simulink model "SF103A_MotRefMdl"  (R2013b)
settings: Solver=FixedStepDiscrete  StartTime=0.0  StopTime=2  FixedStep=.002  RelTol=1e-3
values from neighbouring files (symbols this model uses):
  ARCHGLBPRM_2MILLISEC_SEC_F32 = DataDict.Constant    [SF103A_MotRefMdl_DataDict.m]
  ARCHGLBPRM_2OVERSQRT3_ULS_F32 = DataDict.Constant    [SF103A_MotRefMdl_DataDict.m]
  ARCHGLBPRM_2PI_ULS_F32 = DataDict.Constant    [SF103A_MotRefMdl_DataDict.m]
  ARCHGLBPRM_4OVERSQRT3_ULS_F32 = DataDict.Constant    [SF103A_MotRefMdl_DataDict.m]
  ARCHGLBPRM_5PIOVER4_ULS_F32 = DataDict.Constant    [SF103A_MotRefMdl_DataDict.m]
  ARCHGLBPRM_FLOATZEROTHD_ULS_F32 = DataDict.Constant    [SF103A_MotRefMdl_DataDict.m]
  ARCHGLBPRM_HALFSQRT3_ULS_F32 = DataDict.Constant    [SF103A_MotRefMdl_DataDict.m]
  ARCHGLBPRM_PI_ULS_F32 = DataDict.Constant    [SF103A_MotRefMdl_DataDict.m]
  MotRefMdlCurrDaxBoostGain = DataDict.Calibration    [SF103A_MotRefMdl_DataDict.m]
  MotRefMdlCurrDaxQaxRefDelta = DataDict.Calibration    [SF103A_MotRefMdl_DataDict.m]
  MotRefMdlCurrItrnTolr = DataDict.Calibration    [SF103A_MotRefMdl_DataDict.m]
  MotRefMdlFbCtrlDi = DataDict.Calibration    [SF103A_MotRefMdl_DataDict.m]
  MotRefMdlIvtrDeadTiBrdgVltgSca = DataDict.Calibration    [SF103A_MotRefMdl_DataDict.m]
  MotRefMdlMinCurrItrnLim = DataDict.Calibration    [SF103A_MotRefMdl_DataDict.m]
  MotRefMdlMotCurrDaxMaxSca = DataDict.Calibration    [SF103A_MotRefMdl_DataDict.m]
  MotRefMdlMotVltgDerivtvTiCon = DataDict.Calibration    [SF103A_MotRefMdl_DataDict.m]
  MotRefMdlRefLocnItrnLim = DataDict.Calibration    [SF103A_MotRefMdl_DataDict.m]
  MotRefMdlTqItrnLim = DataDict.Calibration    [SF103A_MotRefMdl_DataDict.m]
  MotRefMdlTqItrnTolr = DataDict.Calibration    [SF103A_MotRefMdl_DataDict.m]
  MotRefMdlVltgModDynCmpEna = DataDict.Calibration    [SF103A_MotRefMdl_DataDict.m]
  MotRefMdlVltgOverRThdSca = DataDict.Calibration    [SF103A_MotRefMdl_DataDict.m]
  SysGlbPrmMotPoleCnt = DataDict.ImprtdCal    [SF103A_MotRefMdl_DataDict.m]
undefined symbols (not defined in the file or in its folder): MotQuad1
libraries: NxtrLim x18, simulink x4, LnrIntrpn x3, Fil x2, NxtrAbslt x2, FixdToFloat x2, FloatToFixd x2, NxtrMath x1
(part 7 of 7)

== system SF103A_MotRefMdl/MotRefMdl/MotRefMdlPer1/LocateTorqueExtremes/WrapBracketAngles/No_Wrapping ==
  note: NOTE: Zero-based indexing
  TqAry : Inport  RequirementInfo={} %GIDa_95b60389_312e_4e00_baea_f2a06bc6961c
  Idx : Inport  RequirementInfo={} %GIDa_85d3ca93_8505_4e13_896f_eb03525bfb00  Port=2
  Action Port : ActionPort  ActionType=else
  Add : Sum  RequirementInfo="{'linktype_rmi_doors' '0000bb42 (/E-STEER Core/SubSystem Specifications/Application Functions/SF99/SF103A Motor Reference Model)' '#SF103A_138' 'true' 'REQ:  SF103A_138' '' } %GIDa_76d2b924_a1a6_47e1_8dc3_f936241e4074"  Inputs=+-
  Add1 : Sum  RequirementInfo="{'linktype_rmi_doors' '0000bb42 (/E-STEER Core/SubSystem Specifications/Application Functions/SF99/SF103A Motor Reference Model)' '#SF103A_138' 'true' 'REQ:  SF103A_138' '' } %GIDa_2d784fd6_0602_4f9b_a025_1580a0ab04f6"
  Bus Creator : BusCreator  RequirementInfo={} %GIDa_72eb0c74_95b4_429b_92eb_e52945b126cd  Inputs=6
  Constant1 : Constant  RequirementInfo="{'linktype_rmi_doors' '0000bb42 (/E-STEER Core/SubSystem Specifications/Application Functions/SF99/SF103A Motor Reference Model)' '#SF103A_138' 'true' 'REQ:  SF103A_138' '' } %GIDa_ebffaea6_e14f_413b_adce_d0d0bfcaa7a2"  SampleTime=-1
  Constant2 : Constant  RequirementInfo="{'linktype_rmi_doors' '0000bb42 (/E-STEER Core/SubSystem Specifications/Application Functions/SF99/SF103A Motor Reference Model)' '#SF103A_138' 'true' 'REQ:  SF103A_138' '' } %GIDa_04d63c2b_3e97_4bb2_a3c0_64e6c76ecc75"  SampleTime=-1
  Constant6 : Constant  RequirementInfo="{'linktype_rmi_doors' '0000bb42 (/E-STEER Core/SubSystem Specifications/Application Functions/SF99/SF103A Motor Reference Model)' '#SF103A_138' 'true' 'REQ:  SF103A_138' '' } %GIDa_7fe1ae96_fb88_4a92_9eeb_3c5b2c10fb83"  Value=MotRefMdlCurrDaxQaxRefDelta
  CopyRight2 : Subsystem  Description=|  mask(Copyright Information){none=on}
      | Copyright info block.                                               
      |                                                                     
      | Place copyright information at the top of every subsystem in design.
      mask prompts: none "No parameters"
      mask help: Place copyright information at the top of every subsystem in design.
      mask Display:
      | NxtrConf = 'Nexteer Confidential';
      | 
      | sys = bdroot; %handle for the current model ("system")
      | first = get_param(sys,'Created');
      | first = first(end-3:end);  %year is last four digits
      | 
      | last = get_param(sys,'LastModifiedDate');
      | if isempty(last)
      |     last = datestr(now,'yyyy');
      | else
      |     last = last(end-3:end);
      | end
      | 
      | if strcmp(first,last)
      |     fprintf('%s -- Copyright %s Nexteer',NxtrConf,first)
      | else
      |     fprintf('%s -- %s%s- %s Nexteer',NxtrConf,char(169),first,last)
      | end
  Index Vector : MultiPortSwitch  RequirementInfo="{'linktype_rmi_doors' '0000bb42 (/E-STEER Core/SubSystem Specifications/Application Functions/SF99/SF103A Motor Reference Model)' '#SF103A_138' 'true' 'REQ:  SF103A_138' '' } %GIDa_7f96635d_e863_42f7_be0b_d83f99408380"  DataPortOrder=Zero-based contiguous  Inputs=1
  Index Vector1 : MultiPortSwitch  RequirementInfo="{'linktype_rmi_doors' '0000bb42 (/E-STEER Core/SubSystem Specifications/Application Functions/SF99/SF103A Motor Reference Model)' '#SF103A_138' 'true' 'REQ:  SF103A_138' '' } %GIDa_df08fecc_11d0_46ed_8f6c_a3725551e30a"  DataPortOrder=Zero-based contiguous  Inputs=1
  Index Vector2 : MultiPortSwitch  RequirementInfo="{'linktype_rmi_doors' '0000bb42 (/E-STEER Core/SubSystem Specifications/Application Functions/SF99/SF103A Motor Reference Model)' '#SF103A_138' 'true' 'REQ:  SF103A_138' '' } %GIDa_93665409_302c_47f3_aba1_ec404b710aa3"  DataPortOrder=Zero-based contiguous  Inputs=1
  Index Vector3 : MultiPortSwitch  RequirementInfo="{'linktype_rmi_doors' '0000bb42 (/E-STEER Core/SubSystem Specifications/Application Functions/SF99/SF103A Motor Reference Model)' '#SF103A_138' 'true' 'REQ:  SF103A_138' '' } %GIDa_c4c60c45_93ef_41e4_9634_c6d7fcea99cf"  DataPortOrder=Zero-based contiguous  Inputs=1
  Index Vector4 : MultiPortSwitch  RequirementInfo="{'linktype_rmi_doors' '0000bb42 (/E-STEER Core/SubSystem Specifications/Application Functions/SF99/SF103A Motor Reference Model)' '#SF103A_138' 'true' 'REQ:  SF103A_138' '' } %GIDa_24382880_2f97_4ce1_8410_907a3d96e683"  DataPortOrder=Zero-based contiguous  Inputs=1
  Index Vector5 : MultiPortSwitch  RequirementInfo="{'linktype_rmi_doors' '0000bb42 (/E-STEER Core/SubSystem Specifications/Application Functions/SF99/SF103A Motor Reference Model)' '#SF103A_138' 'true' 'REQ:  SF103A_138' '' } %GIDa_8818387d_5b6e_4e1f_aee0_609f703e5b56"  DataPortOrder=Zero-based contiguous  Inputs=1
  IntrpnPts : Outport  RequirementInfo={} %GIDa_c42d3cb8_30dc_40e3_b440_084aefa295f6
  wires:
  TqAry/1 -> [torques]
  Idx/1 -> [index]
  Index Vector2/1 -> Bus Creator/1  "UpprDelta"
  Index Vector5/1 -> Bus Creator/2  "UpprTq"
  Index Vector/1 -> Bus Creator/3  "MidDelta"
  Index Vector1/1 -> Bus Creator/4  "MidTq"
  Index Vector3/1 -> Bus Creator/5  "LowrDelta"
  Index Vector4/1 -> Bus Creator/6  "LowrTq"
  Bus Creator/1 -> IntrpnPts/1
  [index] -> Index Vector1/1, Index Vector/1
  [deltas] -> Index Vector/2
  [torques] -> Index Vector1/2
  Add/1 -> Index Vector4/1, Index Vector3/1
  [index] -> Add/1
  [deltas] -> Index Vector3/2
  [torques] -> Index Vector4/2
  Constant2/1 -> Add/2
  Constant6/1 -> [deltas]
  Add1/1 -> Index Vector5/1, Index Vector2/1
  [index] -> Add1/1
  [deltas] -> Index Vector2/2
  [torques] -> Index Vector5/2
  Constant1/1 -> Add1/2

== system SF103A_MotRefMdl/MotRefMdl/MotRefMdlPer1/LocateTorqueExtremes/WrapBracketAngles/Wrap_Lowr ==
  note: Wrap the bracket angles to prevent errors if the peak torque is at an end point of the array.
  note: NOTE: Zero-based indexing
  note: NOTE: Zero-based indexing
  TqAry : Inport  RequirementInfo={} %GIDa_3fa072dd_5fe7_4c7f_8ca0_b3b2c315a3d7
  Idx : Inport  RequirementInfo={} %GIDa_ac2632b2_0763_4a9f_acb0_58eaeea18d90  Port=2
  Action Port : ActionPort  ActionType=then
  Add : Sum  RequirementInfo="{'linktype_rmi_doors' '0000bb42 (/E-STEER Core/SubSystem Specifications/Application Functions/SF99/SF103A Motor Reference Model)' '#SF103A_100' 'true' 'REQ:  SF103A_100' '' } %GIDa_bbfa6807_85b6_4d68_9ac2_192e203651ce"
  Bus Creator : BusCreator  RequirementInfo={} %GIDa_6ae9f6d7_663f_44bb_aed5_5cfe1f01c131  Inputs=6
  Constant10 : Constant  RequirementInfo="{'linktype_rmi_doors' '0000bb42 (/E-STEER Core/SubSystem Specifications/Application Functions/SF99/SF103A Motor Reference Model)' '#SF103A_100' 'true' 'REQ:  SF103A_100' '' } %GIDa_50cc564d_d63d_4f2a_9d9f_cac9422135cc"  Value=ARCHGLBPRM_5PIOVER4_ULS_F32  SampleTime=-1
  Constant2 : Constant  RequirementInfo="{'linktype_rmi_doors' '0000bb42 (/E-STEER Core/SubSystem Specifications/Application Functions/SF99/SF103A Motor Reference Model)' '#SF103A_100' 'true' 'REQ:  SF103A_100' '' } %GIDa_aa06f351_d05b_401f_b871_10ebb36fa07b"  SampleTime=-1
  Constant5 : Constant  RequirementInfo="{'linktype_rmi_doors' '0000bb42 (/E-STEER Core/SubSystem Specifications/Application Functions/SF99/SF103A Motor Reference Model)' '#SF103A_100' 'true' 'REQ:  SF103A_100' '' } %GIDa_ccd9da5e_f0d6_4880_a9e7_d696bf84086b"  Value=7  SampleTime=-1
  Constant6 : Constant  RequirementInfo="{'linktype_rmi_doors' '0000bb42 (/E-STEER Core/SubSystem Specifications/Application Functions/SF99/SF103A Motor Reference Model)' '#SF103A_100' 'true' 'REQ:  SF103A_100' '' } %GIDa_96bf6f88_4e27_4e9c_b012_5186d2ffe8a1"  Value=MotRefMdlCurrDaxQaxRefDelta
  CopyRight2 : Subsystem  Description=|  mask(Copyright Information){none=on}
      | Copyright info block.                                               
      |                                                                     
      | Place copyright information at the top of every subsystem in design.
      mask prompts: none "No parameters"
      mask help: Place copyright information at the top of every subsystem in design.
      mask Display:
      | NxtrConf = 'Nexteer Confidential';
      | 
      | sys = bdroot; %handle for the current model ("system")
      | first = get_param(sys,'Created');
      | first = first(end-3:end);  %year is last four digits
      | 
      | last = get_param(sys,'LastModifiedDate');
      | if isempty(last)
      |     last = datestr(now,'yyyy');
      | else
      |     last = last(end-3:end);
      | end
      | 
      | if strcmp(first,last)
      |     fprintf('%s -- Copyright %s Nexteer',NxtrConf,first)
      | else
      |     fprintf('%s -- %s%s- %s Nexteer',NxtrConf,char(169),first,last)
      | end
  Index Vector : MultiPortSwitch  RequirementInfo="{'linktype_rmi_doors' '0000bb42 (/E-STEER Core/SubSystem Specifications/Application Functions/SF99/SF103A Motor Reference Model)' '#SF103A_100' 'true' 'REQ:  SF103A_100' '' } %GIDa_f284666c_4280_416f_bb28_94f7017bb156"  DataPortOrder=Zero-based contiguous  Inputs=1
  Index Vector1 : MultiPortSwitch  RequirementInfo="{'linktype_rmi_doors' '0000bb42 (/E-STEER Core/SubSystem Specifications/Application Functions/SF99/SF103A Motor Reference Model)' '#SF103A_100' 'true' 'REQ:  SF103A_100' '' } %GIDa_0a60c7cf_ad5b_4d31_b924_ede69bd63232"  DataPortOrder=Zero-based contiguous  Inputs=1
  Index Vector3 : MultiPortSwitch  RequirementInfo="{'linktype_rmi_doors' '0000bb42 (/E-STEER Core/SubSystem Specifications/Application Functions/SF99/SF103A Motor Reference Model)' '#SF103A_100' 'true' 'REQ:  SF103A_100' '' } %GIDa_be7b801b_7061_44d0_9475_e2a0cf41a1f8"  DataPortOrder=Zero-based contiguous  Inputs=1
  Index Vector4 : MultiPortSwitch  RequirementInfo="{'linktype_rmi_doors' '0000bb42 (/E-STEER Core/SubSystem Specifications/Application Functions/SF99/SF103A Motor Reference Model)' '#SF103A_100' 'true' 'REQ:  SF103A_100' '' } %GIDa_6c350bbb_893e_4c96_8400_0beeadbdbe17"  DataPortOrder=Zero-based contiguous  Inputs=1
  Index Vector7 : MultiPortSwitch  RequirementInfo="{'linktype_rmi_doors' '0000bb42 (/E-STEER Core/SubSystem Specifications/Application Functions/SF99/SF103A Motor Reference Model)' '#SF103A_100' 'true' 'REQ:  SF103A_100' '' } %GIDa_519b081d_38f5_4d6a_a715_51094f02bb87"  DataPortOrder=Zero-based contiguous  Inputs=1
  Unary Minus1 : UnaryMinus  RequirementInfo="{'linktype_rmi_doors' '0000bb42 (/E-STEER Core/SubSystem Specifications/Application Functions/SF99/SF103A Motor Reference Model)' '#SF103A_100' 'true' 'REQ:  SF103A_100' '' } %GIDa_9f9d32e8_b716_415d_892e_e7ee7d1e276e"
  IntrpnPts : Outport  RequirementInfo={} %GIDa_19e77f56_d0bb_4149_934f_3a491223ec4d
  wires:
  TqAry/1 -> [torques]
  Idx/1 -> [index]
  Index Vector3/1 -> Bus Creator/1  "UpprDelta"
  Index Vector4/1 -> Bus Creator/2  "UpprTq"
  Index Vector/1 -> Bus Creator/3  "MidDelta"
  Index Vector1/1 -> Bus Creator/4  "MidTq"
  Unary Minus1/1 -> Bus Creator/5  "LowrDelta"
  Index Vector7/1 -> Bus Creator/6  "LowrTq"
  Bus Creator/1 -> IntrpnPts/1
  Constant5/1 -> Index Vector7/1
  [torques] -> Index Vector7/2
  [index] -> Index Vector1/1, Index Vector/1
  [deltas] -> Index Vector/2
  [torques] -> Index Vector1/2
  Add/1 -> Index Vector4/1, Index Vector3/1
  [index] -> Add/1
  [deltas] -> Index Vector3/2
  [torques] -> Index Vector4/2
  Constant2/1 -> Add/2
  Constant6/1 -> [deltas]
  Constant10/1 -> Unary Minus1/1

== system SF103A_MotRefMdl/MotRefMdl/MotRefMdlPer1/LocateTorqueExtremes/WrapBracketAngles/Wrap_Uppr ==
  note: NOTE: Zero-based indexing
  note: NOTE: Zero-based indexing
  note: Wrap the bracket angles to prevent errors if the peak torque is at an end point of the array.
  TqAry : Inport  RequirementInfo={} %GIDa_4e03596c_594b_46a4_893d_3c51f76a8d89
  Idx : Inport  RequirementInfo={} %GIDa_495fed72_a362_426b_a505_cb4884a11291  Port=2
  Action Port : ActionPort  ActionType=elseif
  Add : Sum  RequirementInfo="{'linktype_rmi_doors' '0000bb42 (/E-STEER Core/SubSystem Specifications/Application Functions/SF99/SF103A Motor Reference Model)' '#SF103A_100' 'true' 'REQ:  SF103A_100' '' } %GIDa_e053bb14_2f76_4bb0_9f70_fd6907089663"  Inputs=+-
  Bus Creator : BusCreator  RequirementInfo={} %GIDa_602201cd_6751_4818_8000_e3abdff492eb  Inputs=6
  Constant : Constant  RequirementInfo="{'linktype_rmi_doors' '0000bb42 (/E-STEER Core/SubSystem Specifications/Application Functions/SF99/SF103A Motor Reference Model)' '#SF103A_100' 'true' 'REQ:  SF103A_100' '' } %GIDa_154c60c8_e670_4a5e_b123_a8ddfb972f0f"  Value=ARCHGLBPRM_PI_ULS_F32  SampleTime=-1
  Constant1 : Constant  RequirementInfo="{'linktype_rmi_doors' '0000bb42 (/E-STEER Core/SubSystem Specifications/Application Functions/SF99/SF103A Motor Reference Model)' '#SF103A_100' 'true' 'REQ:  SF103A_100' '' } %GIDa_9bb1aafd_43ae_47b8_94bb_0eb28064f111"  Value=0  SampleTime=-1
  Constant2 : Constant  RequirementInfo="{'linktype_rmi_doors' '0000bb42 (/E-STEER Core/SubSystem Specifications/Application Functions/SF99/SF103A Motor Reference Model)' '#SF103A_100' 'true' 'REQ:  SF103A_100' '' } %GIDa_b92fae25_25fa_4196_9949_c384a6bb8643"  SampleTime=-1
  Constant6 : Constant  RequirementInfo="{'linktype_rmi_doors' '0000bb42 (/E-STEER Core/SubSystem Specifications/Application Functions/SF99/SF103A Motor Reference Model)' '#SF103A_100' 'true' 'REQ:  SF103A_100' '' } %GIDa_d45d87cc_3c8d_434a_9d9f_0536981e822a"  Value=MotRefMdlCurrDaxQaxRefDelta
  CopyRight2 : Subsystem  Description=|  mask(Copyright Information){none=on}
      | Copyright info block.                                               
      |                                                                     
      | Place copyright information at the top of every subsystem in design.
      mask prompts: none "No parameters"
      mask help: Place copyright information at the top of every subsystem in design.
      mask Display:
      | NxtrConf = 'Nexteer Confidential';
      | 
      | sys = bdroot; %handle for the current model ("system")
      | first = get_param(sys,'Created');
      | first = first(end-3:end);  %year is last four digits
      | 
      | last = get_param(sys,'LastModifiedDate');
      | if isempty(last)
      |     last = datestr(now,'yyyy');
      | else
      |     last = last(end-3:end);
      | end
      | 
      | if strcmp(first,last)
      |     fprintf('%s -- Copyright %s Nexteer',NxtrConf,first)
      | else
      |     fprintf('%s -- %s%s- %s Nexteer',NxtrConf,char(169),first,last)
      | end
  Index Vector : MultiPortSwitch  RequirementInfo="{'linktype_rmi_doors' '0000bb42 (/E-STEER Core/SubSystem Specifications/Application Functions/SF99/SF103A Motor Reference Model)' '#SF103A_100' 'true' 'REQ:  SF103A_100' '' } %GIDa_375a72ea_af8b_433e_b0af_75ca9819e517"  DataPortOrder=Zero-based contiguous  Inputs=1
  Index Vector1 : MultiPortSwitch  RequirementInfo="{'linktype_rmi_doors' '0000bb42 (/E-STEER Core/SubSystem Specifications/Application Functions/SF99/SF103A Motor Reference Model)' '#SF103A_100' 'true' 'REQ:  SF103A_100' '' } %GIDa_e36d34d9_7f06_4e66_a2a1_2b1341b8f2a4"  DataPortOrder=Zero-based contiguous  Inputs=1
  Index Vector2 : MultiPortSwitch  RequirementInfo="{'linktype_rmi_doors' '0000bb42 (/E-STEER Core/SubSystem Specifications/Application Functions/SF99/SF103A Motor Reference Model)' '#SF103A_100' 'true' 'REQ:  SF103A_100' '' } %GIDa_1838deb4_a05c_4d2f_9cfa_2fa6ae4e7b0c"  DataPortOrder=Zero-based contiguous  Inputs=1
  Index Vector3 : MultiPortSwitch  RequirementInfo="{'linktype_rmi_doors' '0000bb42 (/E-STEER Core/SubSystem Specifications/Application Functions/SF99/SF103A Motor Reference Model)' '#SF103A_100' 'true' 'REQ:  SF103A_100' '' } %GIDa_0c1b0eb8_45d1_4317_a22f_d08019f0e40c"  DataPortOrder=Zero-based contiguous  Inputs=1
  Index Vector4 : MultiPortSwitch  RequirementInfo="{'linktype_rmi_doors' '0000bb42 (/E-STEER Core/SubSystem Specifications/Application Functions/SF99/SF103A Motor Reference Model)' '#SF103A_100' 'true' 'REQ:  SF103A_100' '' } %GIDa_fe3aa5e1_87ea_423f_a2cb_7e97908e5fd6"  DataPortOrder=Zero-based contiguous  Inputs=1
  IntrpnPts : Outport  RequirementInfo={} %GIDa_8903bef9_e454_47cd_a8dc_61025ef2e460
  wires:
  TqAry/1 -> [torques]
  Idx/1 -> [index]
  Constant/1 -> Bus Creator/1  "UpprDelta"
  Index Vector2/1 -> Bus Creator/2  "UpprTq"
  Index Vector/1 -> Bus Creator/3  "MidDelta"
  Index Vector1/1 -> Bus Creator/4  "MidTq"
  Index Vector3/1 -> Bus Creator/5  "LowrDelta"
  Index Vector4/1 -> Bus Creator/6  "LowrTq"
  Bus Creator/1 -> IntrpnPts/1
  [index] -> Index Vector1/1, Index Vector/1
  [deltas] -> Index Vector/2
  [torques] -> Index Vector1/2
  Add/1 -> Index Vector4/1, Index Vector3/1
  [index] -> Add/1
  [deltas] -> Index Vector3/2
  [torques] -> Index Vector4/2
  Constant2/1 -> Add/2
  Constant1/1 -> Index Vector2/1
  [torques] -> Index Vector2/2
  Constant6/1 -> [deltas]

== system SF103A_MotRefMdl/MotRefMdl/MotRefMdlPer1/MotCurrAg_AlphaCalc/Wrap Angle/CopyRight2 ==

== system SF103A_MotRefMdl/MotRefMdl/MotRefMdlPer1/VoltageScheduling/If Action Subsystem/CopyRight2 ==

== system SF103A_MotRefMdl/MotRefMdl/MotRefMdlPer1/VoltageScheduling/If Action Subsystem1/CopyRight2 ==

== system SF103A_MotRefMdl/MotRefMdl/MotRefMdlPer1/CalcMinimumMotorCurrent/WhileIteratorSubsystem/F_ParabolicInterpolation/If Action Subsystem ==
  Num : Inport
  Den : Inport  Port=2
  Idx2 : Inport  Port=3
  Action Port : ActionPort  ActionType=then
  Add : Sum
  Divide : Product  Inputs=*/
  Out1 : Outport
  wires:
  Num/1 -> Divide/1
  Den/1 -> Divide/2
  Divide/1 -> Add/1
  Idx2/1 -> Add/2
  Add/1 -> Out1/1

== system SF103A_MotRefMdl/MotRefMdl/MotRefMdlPer1/CalcMinimumMotorCurrent/WhileIteratorSubsystem/F_ParabolicInterpolation/If Action Subsystem1 ==
  In1 : Inport
  Action Port : ActionPort  ActionType=else
  Out1 : Outport
  wires:
  In1/1 -> Out1/1

== system SF103A_MotRefMdl/MotRefMdl/MotRefMdlPer1/CalcMinimumMotorCurrent/WhileIteratorSubsystem/Refine_Higher/CopyRight2 ==

== system SF103A_MotRefMdl/MotRefMdl/MotRefMdlPer1/CalcMinimumMotorCurrent/WhileIteratorSubsystem/Refine_Lower/CopyRight2 ==

== system SF103A_MotRefMdl/MotRefMdl/MotRefMdlPer1/DAxisCurrentBoost/If Action Subsystem/If Action Subsystem/CopyRight2 ==

== system SF103A_MotRefMdl/MotRefMdl/MotRefMdlPer1/DAxisCurrentBoost/If Action Subsystem/If Action Subsystem/If Action Subsystem ==
  BoostProposed : Inport  RequirementInfo={} %GIDa_10e66d27_4695_4469_a1da_4ba30e5da203
  Action Port : ActionPort  ActionType=then
  CopyRight2 : Subsystem  Description=|  mask(Copyright Information){none=on}
      | Copyright info block.                                               
      |                                                                     
      | Place copyright information at the top of every subsystem in design.
      mask prompts: none "No parameters"
      mask help: Place copyright information at the top of every subsystem in design.
      mask Display:
      | NxtrConf = 'Nexteer Confidential';
      | 
      | sys = bdroot; %handle for the current model ("system")
      | first = get_param(sys,'Created');
      | first = first(end-3:end);  %year is last four digits
      | 
      | last = get_param(sys,'LastModifiedDate');
      | if isempty(last)
      |     last = datestr(now,'yyyy');
      | else
      |     last = last(end-3:end);
      | end
      | 
      | if strcmp(first,last)
      |     fprintf('%s -- Copyright %s Nexteer',NxtrConf,first)
      | else
      |     fprintf('%s -- %s%s- %s Nexteer',NxtrConf,char(169),first,last)
      | end
  CurrDaxBoostd : Outport  RequirementInfo={} %GIDa_54fbdd4a_e87d_4384_8e62_630c1893f799
  wires:
  BoostProposed/1 -> CurrDaxBoostd/1

== system SF103A_MotRefMdl/MotRefMdl/MotRefMdlPer1/DAxisCurrentBoost/If Action Subsystem/If Action Subsystem/If Action Subsystem1 ==
  CurrDaxAtPeakTq : Inport  RequirementInfo={} %GIDa_ddb806f7_84df_4424_9ff4_e056cb738e7a
  Action Port : ActionPort  ActionType=else
  CopyRight2 : Subsystem  Description=|  mask(Copyright Information){none=on}
      | Copyright info block.                                               
      |                                                                     
      | Place copyright information at the top of every subsystem in design.
      mask prompts: none "No parameters"
      mask help: Place copyright information at the top of every subsystem in design.
      mask Display:
      | NxtrConf = 'Nexteer Confidential';
      | 
      | sys = bdroot; %handle for the current model ("system")
      | first = get_param(sys,'Created');
      | first = first(end-3:end);  %year is last four digits
      | 
      | last = get_param(sys,'LastModifiedDate');
      | if isempty(last)
      |     last = datestr(now,'yyyy');
      | else
      |     last = last(end-3:end);
      | end
      | 
      | if strcmp(first,last)
      |     fprintf('%s -- Copyright %s Nexteer',NxtrConf,first)
      | else
      |     fprintf('%s -- %s%s- %s Nexteer',NxtrConf,char(169),first,last)
      | end
  CurrDaxBoostd : Outport  RequirementInfo={} %GIDa_10be653f_eba4_4d66_b27a_557773872142
  wires:
  CurrDaxAtPeakTq/1 -> CurrDaxBoostd/1

== system SF103A_MotRefMdl/MotRefMdl/MotRefMdlPer1/LocateRef/for_loop_stuff_here/For Iterator Subsystem/CopyRight2 ==

== system SF103A_MotRefMdl/MotRefMdl/MotRefMdlPer1/LocateRef/for_loop_stuff_here/For Iterator Subsystem/CurrToVoltTest ==
  note: Logic in model matches EA3 code implementation.
      | Equivalent logic to requirements.  IF A >=B THEN true, vs. IF A<B THEN false
  IdRef_Amp : Inport  RequirementInfo={} %GIDa_ce9658aa_217e_4ea6_9ad8_48fb9230f3de
  IqRef_Amp : Inport  RequirementInfo={} %GIDa_590e4f02_27d3_4430_a621_d5f2b0116d0f  Port=2
  InterCalcns : Inport  RequirementInfo={} %GIDa_f44b55eb_ff8d_41d3_b576_1b36bcae7a06  Port=3
  Add : Sum  RequirementInfo="{'linktype_rmi_doors' '0000bb42 (/E-STEER Core/SubSystem Specifications/Application Functions/SF99/SF103A Motor Reference Model)' '#SF103A_116' 'true' 'REQ:  SF103A_116' '' } %GIDa_b7e2bd32_b25a_4e68_9597_585732479309"  Inputs=+++
  Add1 : Sum  RequirementInfo="{'linktype_rmi_doors' '0000bb42 (/E-STEER Core/SubSystem Specifications/Application Functions/SF99/SF103A Motor Reference Model)' '#SF103A_125' 'true' 'REQ:  SF103A_125' '' } %GIDa_148dbd96_bb79_4487_948d_1faa9b0a8dd7"
  Bus Selector2 : BusSelector  RequirementInfo={} %GIDa_58fe1b81_d674_4d59_a357_9313fbf42842  OutputSignals=ReacncQaxOverR,ReacncDaxOverR,EgOverR_Ampr,VovrRAllSqd_AmprSqd
  CopyRight2 : Subsystem  Description=|  mask(Copyright Information){none=on}
      | Copyright info block.                                               
      |                                                                     
      | Place copyright information at the top of every subsystem in design.
      mask prompts: none "No parameters"
      mask help: Place copyright information at the top of every subsystem in design.
      mask Display:
      | NxtrConf = 'Nexteer Confidential';
      | 
      | sys = bdroot; %handle for the current model ("system")
      | first = get_param(sys,'Created');
      | first = first(end-3:end);  %year is last four digits
      | 
      | last = get_param(sys,'LastModifiedDate');
      | if isempty(last)
      |     last = datestr(now,'yyyy');
      | else
      |     last = last(end-3:end);
      | end
      | 
      | if strcmp(first,last)
      |     fprintf('%s -- Copyright %s Nexteer',NxtrConf,first)
      | else
      |     fprintf('%s -- %s%s- %s Nexteer',NxtrConf,char(169),first,last)
      | end
  FALSE1 : Constant  RequirementInfo="{'linktype_rmi_doors' '0000bb42 (/E-STEER Core/SubSystem Specifications/Application Functions/SF99/SF103A Motor Reference Model)' '#SF103A_125' 'true' 'REQ:  SF103A_125' '' } %GIDa_f2df8fef_5195_43ac_8889_d13281d10792"  Value=false  OutDataTypeStr=boolean
  FALSE2 : Constant  RequirementInfo="{'linktype_rmi_doors' '0000bb42 (/E-STEER Core/SubSystem Specifications/Application Functions/SF99/SF103A Motor Reference Model)' '#SF103A_125' 'true' 'REQ:  SF103A_125' '' } %GIDa_f6784742_eefe_468d_8b76_246ef0e2a438"  Value=true  OutDataTypeStr=boolean
  If1 : If  RequirementInfo="{'linktype_rmi_doors' '0000bb42 (/E-STEER Core/SubSystem Specifications/Application Functions/SF99/SF103A Motor Reference Model)' '#SF103A_125' 'true' 'REQ:  SF103A_125' '' } %GIDa_e6459d24_2539_4aa4_9bf7_e15cfc62054d"  NumInputs=2  IfExpression=u1 < u2
  Math Function : Math  RequirementInfo="{'linktype_rmi_doors' '0000bb42 (/E-STEER Core/SubSystem Specifications/Application Functions/SF99/SF103A Motor Reference Model)' '#SF103A_125' 'true' 'REQ:  SF103A_125' '' } %GIDa_a41b84f2_f4bc_43cc_a211_88336ca9d4a8"  Operator=square  SaturateOnIntegerOverflow=on
  Math Function1 : Math  RequirementInfo="{'linktype_rmi_doors' '0000bb42 (/E-STEER Core/SubSystem Specifications/Application Functions/SF99/SF103A Motor Reference Model)' '#SF103A_125' 'true' 'REQ:  SF103A_125' '' } %GIDa_e1d91394_7358_4c48_a31d_c4d31a4b7844"  Operator=square  SaturateOnIntegerOverflow=on
  Merge : Merge  RequirementInfo="{'linktype_rmi_doors' '0000bb42 (/E-STEER Core/SubSystem Specifications/Application Functions/SF99/SF103A Motor Reference Model)' '#SF103A_125' 'true' 'REQ:  SF103A_125' '' } %GIDa_5aca2e4b_fa43_40a7_9e0d_4ee5ab088903"
  Product : Product  RequirementInfo="{'linktype_rmi_doors' '0000bb42 (/E-STEER Core/SubSystem Specifications/Application Functions/SF99/SF103A Motor Reference Model)' '#SF103A_116' 'true' 'REQ:  SF103A_116' '' } %GIDa_a7c1ed44_b973_47c9_83af_058c526982c4"  RndMeth=Zero
  Product1 : Product  RequirementInfo="{'linktype_rmi_doors' '0000bb42 (/E-STEER Core/SubSystem Specifications/Application Functions/SF99/SF103A Motor Reference Model)' '#SF103A_116' 'true' 'REQ:  SF103A_116' '' } %GIDa_7b3606b5_1b3b_4f3c_b9b7_5eed9f0f75e9"  RndMeth=Zero
  Subtract1 : Sum  RequirementInfo="{'linktype_rmi_doors' '0000bb42 (/E-STEER Core/SubSystem Specifications/Application Functions/SF99/SF103A Motor Reference Model)' '#SF103A_116' 'true' 'REQ:  SF103A_116' '' } %GIDa_ff9c1c17_8b6e_480e_affc_f63c7b3e0c34"  Inputs=+-
  set_false : Subsystem  RequirementInfo="{'linktype_rmi_doors' '0000bb42 (/E-STEER Core/SubSystem Specifications/Application Functions/SF99/SF103A Motor Reference Model)' '#SF103A_125' 'true' 'REQ:  SF103A_125' '' } %GIDa_26f458c7_886d_4114_b7d0_32624bbb92b6"  TreatAsAtomicUnit=on
  set_true : Subsystem  RequirementInfo="{'linktype_rmi_doors' '0000bb42 (/E-STEER Core/SubSystem Specifications/Application Functions/SF99/SF103A Motor Reference Model)' '#SF103A_125' 'true' 'REQ:  SF103A_125' '' } %GIDa_5aa1b058_dadd_4c8b_b0a5_53d417f3faed"  TreatAsAtomicUnit=on
  VoltTest_lgc : Outport  RequirementInfo={} %GIDa_3978efca_b99c_4460_8d64_fa28db9c441c
  VdR : Outport  RequirementInfo={} %GIDa_1adfd60b_8f11_4ed6_a01b_fb2187ed9f1a  Port=2
  VqR : Outport  RequirementInfo={} %GIDa_00042128_9a26_47b3_b780_274c006db6fc  Port=3
  wires:
  Bus Selector2/4 -> If1/2  "<VovrRAllSqd_AmprSqd>"
  Subtract1/1 -> VdR/1, Math Function/1  "VdRTemp_Amp"
  Add/1 -> VqR/1, Math Function1/1  "VqRTemp_Amp"
  Math Function/1 -> Add1/1
  Math Function1/1 -> Add1/2
  Add1/1 -> If1/1
  Merge/1 -> VoltTest_lgc/1
  IqRef_Amp/1 -> Add/1, Product/1
  IdRef_Amp/1 -> Product1/1, Subtract1/2
  InterCalcns/1 -> Bus Selector2/1
  Bus Selector2/1 -> Product/2  "<ReacncQaxOverR>"
  Bus Selector2/2 -> Product1/2  "<ReacncDaxOverR>"
  Bus Selector2/3 -> Add/3  "<EgOverR_Ampr>"
  Product/1 -> Subtract1/1
  Product1/1 -> Add/2
  If1/1 -> set_false/Action
  If1/2 -> set_true/Action
  FALSE1/1 -> set_false/1(In1)
  FALSE2/1 -> set_true/1(In1)
  set_false/1(Out1) -> Merge/1
  set_true/1(Out1) -> Merge/2

== system SF103A_MotRefMdl/MotRefMdl/MotRefMdlPer1/LocateRef/for_loop_stuff_here/For Iterator Subsystem/F_CalcIqCmd_3 ==
  MotTqCmd : Inport
  IdRef_in : Inport  Port=2
  InterCalcns : Inport  Port=3
  Add : Sum
  Bus Selector : BusSelector  OutputSignals=Ke_VoltPerRadPerSec,RelncTqCoeff_Henry_f32
  CopyRight2 : Subsystem  Description=|  mask(Copyright Information){none=on}
      | Copyright info block.                                               
      |                                                                     
      | Place copyright information at the top of every subsystem in design.
      mask prompts: none "No parameters"
      mask help: Place copyright information at the top of every subsystem in design.
      mask Display:
      | NxtrConf = 'Nexteer Confidential';
      | 
      | sys = bdroot; %handle for the current model ("system")
      | first = get_param(sys,'Created');
      | first = first(end-3:end);  %year is last four digits
      | 
      | last = get_param(sys,'LastModifiedDate');
      | if isempty(last)
      |     last = datestr(now,'yyyy');
      | else
      |     last = last(end-3:end);
      | end
      | 
      | if strcmp(first,last)
      |     fprintf('%s -- Copyright %s Nexteer',NxtrConf,first)
      | else
      |     fprintf('%s -- %s%s- %s Nexteer',NxtrConf,char(169),first,last)
      | end
  Product : Product  RndMeth=Zero
  Product1 : Product  Inputs=*/  RndMeth=Zero
  IqRef : Outport
  wires:
  Product1/1 -> IqRef/1
  MotTqCmd/1 -> Product1/1
  Add/1 -> Product1/2
  Bus Selector/1 -> Add/1  "<Ke_VoltPerRadPerSec>"
  IdRef_in/1 -> Product/2
  Bus Selector/2 -> Product/1  "<RelncTqCoeff_Henry_f32>"
  InterCalcns/1 -> Bus Selector/1
  Product/1 -> Add/2

== system SF103A_MotRefMdl/MotRefMdl/MotRefMdlPer1/LocateRef/for_loop_stuff_here/For Iterator Subsystem/If Action Subsystem ==
  In1 : Inport
  In2 : Inport  Port=2
  Action Port : ActionPort  ActionType=then
  Out1 : Outport
  Out2 : Outport  Port=2
  wires:
  In1/1 -> Out1/1
  In2/1 -> Out2/1

== system SF103A_MotRefMdl/MotRefMdl/MotRefMdlPer1/LocateRef/for_loop_stuff_here/For Iterator Subsystem/If Action Subsystem1 ==
  In1 : Inport
  In2 : Inport  Port=2
  Action Port : ActionPort  ActionType=else
  Out1 : Outport
  Out2 : Outport  Port=2
  wires:
  In1/1 -> Out1/1
  In2/1 -> Out2/1

== system SF103A_MotRefMdl/MotRefMdl/MotRefMdlPer1/LocateRef/for_loop_stuff_here/For Iterator Subsystem/use_incoming_values ==
  In1 : Inport
  In2 : Inport  Port=2
  Action Port : ActionPort  ActionType=else
  Out1 : Outport
  Out2 : Outport  Port=2
  wires:
  In1/1 -> Out1/1
  In2/1 -> Out2/1

== system SF103A_MotRefMdl/MotRefMdl/MotRefMdlPer1/LocateRef/for_loop_stuff_here/For Iterator Subsystem/use_new_values ==
  In1 : Inport
  In2 : Inport  Port=2
  Action Port : ActionPort  ActionType=then
  Out1 : Outport
  Out2 : Outport  Port=2
  wires:
  In1/1 -> Out1/1
  In2/1 -> Out2/1

== system SF103A_MotRefMdl/MotRefMdl/MotRefMdlPer1/LocateTorqueExtremes/InterpolatePeakTorque/F_CalculateTorque/CopyRight2 ==

== system SF103A_MotRefMdl/MotRefMdl/MotRefMdlPer1/LocateTorqueExtremes/InterpolatePeakTorque/F_ParabolicInterpolation/CopyRight2 ==

== system SF103A_MotRefMdl/MotRefMdl/MotRefMdlPer1/LocateTorqueExtremes/InterpolatePeakTorque/F_ParabolicInterpolation/If Action Subsystem ==
  Num : Inport
  Den : Inport  Port=2
  Idx2 : Inport  Port=3
  Action Port : ActionPort  ActionType=then
  Add : Sum
  Divide : Product  Inputs=*/
  Out1 : Outport
  wires:
  Num/1 -> Divide/1
  Den/1 -> Divide/2
  Divide/1 -> Add/1
  Idx2/1 -> Add/2
  Add/1 -> Out1/1

== system SF103A_MotRefMdl/MotRefMdl/MotRefMdlPer1/LocateTorqueExtremes/InterpolatePeakTorque/F_ParabolicInterpolation/If Action Subsystem1 ==
  In1 : Inport
  Action Port : ActionPort  ActionType=else
  Out1 : Outport
  wires:
  In1/1 -> Out1/1

== system SF103A_MotRefMdl/MotRefMdl/MotRefMdlPer1/LocateTorqueExtremes/InterpolatePeakTorque/F_VSinCosToIdIq/CopyRight2 ==

== system SF103A_MotRefMdl/MotRefMdl/MotRefMdlPer1/LocateTorqueExtremes/InterpolatePeakTorque/Refine_Higher/CopyRight2 ==

== system SF103A_MotRefMdl/MotRefMdl/MotRefMdlPer1/LocateTorqueExtremes/InterpolatePeakTorque/Refine_Lower/CopyRight2 ==

== system SF103A_MotRefMdl/MotRefMdl/MotRefMdlPer1/LocateTorqueExtremes/Negative/For Iterator Subsystem/CopyRight2 ==

== system SF103A_MotRefMdl/MotRefMdl/MotRefMdlPer1/LocateTorqueExtremes/Negative/For Iterator Subsystem/Found_New_Min ==
  Idx : Inport
  Tq : Inport  Port=2
  Action Port : ActionPort  ActionType=then
  IdxSt : Outport
  TqSt : Outport  Port=2
  wires:
  Tq/1 -> TqSt/1
  Idx/1 -> IdxSt/1

== system SF103A_MotRefMdl/MotRefMdl/MotRefMdlPer1/LocateTorqueExtremes/Positive/For Iterator Subsystem/CopyRight2 ==

== system SF103A_MotRefMdl/MotRefMdl/MotRefMdlPer1/LocateTorqueExtremes/Positive/For Iterator Subsystem/Found_New_Max ==
  Idx : Inport
  Tq : Inport  Port=2
  Action Port : ActionPort  ActionType=then
  IdxSt : Outport
  TqSt : Outport  Port=2
  wires:
  Tq/1 -> TqSt/1
  Idx/1 -> IdxSt/1

== system SF103A_MotRefMdl/MotRefMdl/MotRefMdlPer1/LocateTorqueExtremes/WrapBracketAngles/No_Wrapping/CopyRight2 ==

== system SF103A_MotRefMdl/MotRefMdl/MotRefMdlPer1/LocateTorqueExtremes/WrapBracketAngles/Wrap_Lowr/CopyRight2 ==

== system SF103A_MotRefMdl/MotRefMdl/MotRefMdlPer1/LocateTorqueExtremes/WrapBracketAngles/Wrap_Uppr/CopyRight2 ==

== system SF103A_MotRefMdl/MotRefMdl/MotRefMdlPer1/DAxisCurrentBoost/If Action Subsystem/If Action Subsystem/If Action Subsystem/CopyRight2 ==

== system SF103A_MotRefMdl/MotRefMdl/MotRefMdlPer1/DAxisCurrentBoost/If Action Subsystem/If Action Subsystem/If Action Subsystem1/CopyRight2 ==

== system SF103A_MotRefMdl/MotRefMdl/MotRefMdlPer1/LocateRef/for_loop_stuff_here/For Iterator Subsystem/CurrToVoltTest/CopyRight2 ==

== system SF103A_MotRefMdl/MotRefMdl/MotRefMdlPer1/LocateRef/for_loop_stuff_here/For Iterator Subsystem/CurrToVoltTest/set_false ==
  In1 : Inport
  Action Port : ActionPort  ActionType=then
  Out1 : Outport
  wires:
  In1/1 -> Out1/1

== system SF103A_MotRefMdl/MotRefMdl/MotRefMdlPer1/LocateRef/for_loop_stuff_here/For Iterator Subsystem/CurrToVoltTest/set_true ==
  In1 : Inport
  Action Port : ActionPort  ActionType=else
  Out1 : Outport
  wires:
  In1/1 -> Out1/1

== system SF103A_MotRefMdl/MotRefMdl/MotRefMdlPer1/LocateRef/for_loop_stuff_here/For Iterator Subsystem/F_CalcIqCmd_3/CopyRight2 ==
